simulink model "WiperSystem"  (R2023a)
settings: Solver=FixedStepDiscrete  StartTime=0.0  StopTime=50  RelTol=1e-3  EnableMultiTasking=on
libraries: simulink x1
settings Model: Creator=Ahmed  LastModifiedBy=Ahmed
settings DataIOCC: SaveOutput=off  SaveTime=off
settings OptimizationCC: DefaultParameterBehavior=Inlined  UseDivisionForNetSlopeComputation=on  GainParamInheritBuiltInType=on  UseFloatMulNetSlope=on  InlineInvariantSignals=on  PassReuseOutputArgsAs=Individual arguments  ZeroExternalMemoryAtStartup=off  ZeroInternalMemoryAtStartup=off  NoFixptDivByZeroProtection=on  EfficientFloat2IntCast=on  LifeSpan=1  OptimizeBlockOrder=speed  DifferentSizesBufferReuse=on  EfficientTunableParamExpr=on
settings DebuggingCC: ParameterPrecisionLossMsg=none  ParameterTunabilityLossMsg=error
settings HardwareCC: ProdBitPerPointer=32  ProdBitPerSizeT=32  ProdBitPerPtrDiffT=32  ProdLargestAtomicInteger=Long  ProdLargestAtomicFloat=Double  ProdWordSize=32  ProdLongLongMode=on  ProdHWDeviceType=ARM Compatible->ARM Cortex-M
settings ModelReferenceCC: ModelReferenceNumInstancesAllowed=Single
settings SFSimCC: MATLABDynamicMemAlloc=off
settings RTWCC: Description=Embedded Coder  SystemTargetFile=ert.tlc  GenCodeOnly=on  TemplateMakefile=ert_default_tmf
settings CodeAppCC: ForceParamTrailComments=on  IgnoreCustomStorageClasses=off  OperatorAnnotations=on  SimulinkDataObjDesc=on  SFDataObjDesc=on  CustomSymbolStrGlobalVar=rt$N$M  CustomSymbolStrType=$N$M  CustomSymbolStrFcn=$N$M$F  CustomSymbolStrMacro=$N$M  InsertBlockDesc=on
settings ERTTargetCC: TargetLangStandard=C99 (ISO)  GenerateSampleERTMain=on  IncludeMdlTerminateFcn=off  CombineSignalStateStructs=on  SupportComplex=off  SupportNonInlinedSFcns=on  InlinedParameterPlacement=NonHierarchical  ERTCustomFileTemplate=example_file_process.tlc  ERTFilePackagingFormat=CompactWithDataFile

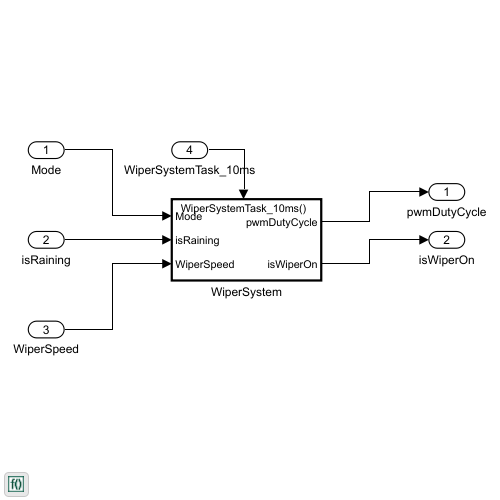
[thumbnail: Simulink's stored preview of the top-level diagram]
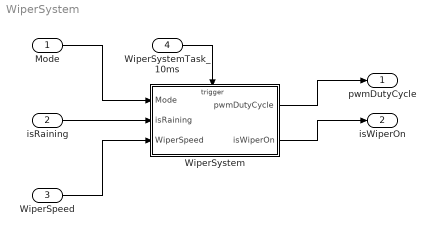
== system WiperSystem ==
  Mode : Inport  OutDataTypeStr=uint8  PortDimensions=1
  isRaining : Inport  Port=2  OutDataTypeStr=boolean  PortDimensions=1
  WiperSpeed : Inport  Port=3  OutDataTypeStr=uint8  PortDimensions=1
  WiperSystemTask_10ms : Inport  Port=4  PortDimensions=1  OutputFunctionCall=on
  WiperSystem : Subsystem  TreatAsAtomicUnit=on
  pwmDutyCycle : Outport  OutDataTypeStr=single  PortDimensions=1
  isWiperOn : Outport  Port=2  OutDataTypeStr=boolean  PortDimensions=1
  wires:
  Mode/1 -> WiperSystem/1(Mode)
  isRaining/1 -> WiperSystem/2(isRaining)
  WiperSpeed/1 -> WiperSystem/3(WiperSpeed)
  WiperSystem/1(pwmDutyCycle) -> pwmDutyCycle/1
  WiperSystem/2(isWiperOn) -> isWiperOn/1
  WiperSystemTask_10ms/1 -> WiperSystem/Trigger

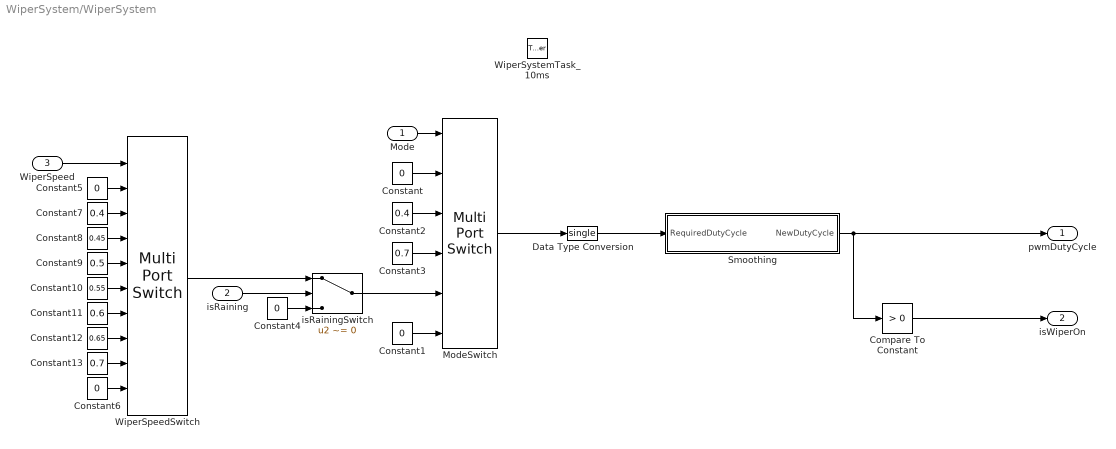
== system WiperSystem/WiperSystem ==
  Mode : Inport
  isRaining : Inport  Port=2
  WiperSpeed : Inport  Port=3
  WiperSystemTask_10ms : TriggerPort  TriggerType=function-call  VariantControl=(inherit)
  Compare To Constant : simulink/Logic and Bit Operations/Compare To Constant  relop=>  const=0  OutDataTypeStr=boolean
  Constant{,1,4..6} (5 alike) : Constant  Value=0
  Constant10 : Constant  Value=0.55
  Constant11 : Constant  Value=0.6
  Constant12 : Constant  Value=0.65
  Constant13 : Constant  Value=0.7
  Constant2 : Constant  Value=0.4
  Constant3 : Constant  Value=0.7
  Constant7 : Constant  Value=0.4
  Constant8 : Constant  Value=0.45
  Constant9 : Constant  Value=0.5
  Data Type Conversion : DataTypeConversion  OutDataTypeStr=single  SaturateOnIntegerOverflow=off  RndMeth=Floor
  ModeSwitch : MultiPortSwitch  DataPortOrder=Zero-based contiguous  Inputs=4  DataPortForDefault=Additional data port  DiagnosticForDefault=None  zeroidx=on  SaturateOnIntegerOverflow=off  InputSameDT=off
  Smoothing : Subsystem
  WiperSpeedSwitch : MultiPortSwitch  DataPortOrder=Zero-based contiguous  Inputs=8  DataPortForDefault=Additional data port  DiagnosticForDefault=None  zeroidx=on  SaturateOnIntegerOverflow=off  InputSameDT=off
  isRainingSwitch : Switch  Criteria=u2 ~= 0  SaturateOnIntegerOverflow=off  InputSameDT=off
  pwmDutyCycle : Outport
  isWiperOn : Outport  Port=2
  wires:
  Compare To Constant/1 -> isWiperOn/1
  Data Type Conversion/1 -> Smoothing/1(RequiredDutyCycle)
  Smoothing/1(NewDutyCycle) -> pwmDutyCycle/1, Compare To Constant/1
  ModeSwitch/1 -> Data Type Conversion/1
  Constant13/1 -> WiperSpeedSwitch/9
  Constant12/1 -> WiperSpeedSwitch/8
  Constant11/1 -> WiperSpeedSwitch/7
  Constant10/1 -> WiperSpeedSwitch/6
  Constant9/1 -> WiperSpeedSwitch/5
  Constant8/1 -> WiperSpeedSwitch/4
  Constant7/1 -> WiperSpeedSwitch/3
  Constant5/1 -> WiperSpeedSwitch/2
  WiperSpeedSwitch/1 -> isRainingSwitch/1
  isRainingSwitch/1 -> ModeSwitch/5
  WiperSpeed/1 -> WiperSpeedSwitch/1
  Constant6/1 -> WiperSpeedSwitch/10
  Constant4/1 -> isRainingSwitch/3
  isRaining/1 -> isRainingSwitch/2
  Constant3/1 -> ModeSwitch/4
  Constant2/1 -> ModeSwitch/3
  Constant1/1 -> ModeSwitch/6
  Constant/1 -> ModeSwitch/2
  Mode/1 -> ModeSwitch/1

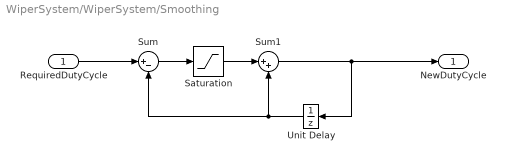
== system WiperSystem/WiperSystem/Smoothing ==
  RequiredDutyCycle : Inport
  Saturation : Saturate  UpperLimit=0.0025  LowerLimit=-0.0025
  Sum : Sum  Inputs=|+-
  Sum1 : Sum  Inputs=|++
  Unit Delay : UnitDelay  SampleTime=-1  HasFrameUpgradeWarning=on
  NewDutyCycle : Outport
  wires:
  RequiredDutyCycle/1 -> Sum/1
  Sum/1 -> Saturation/1
  Saturation/1 -> Sum1/1
  Sum1/1 -> Unit Delay/1, NewDutyCycle/1
  Unit Delay/1 -> Sum1/2, Sum/2
